simulink model "drives_project"  (R2023b)
settings: Solver=VariableStepAuto  StartTime=0.0  StopTime=0.1  RelTol=1e-3
InitFcn:
  | vm=220;
  | f=50;
  | P=2;
  | we=2*pi*f;
  | rs=0.1;
  | lls=0.06;
  | rr=0.1
  | llr=0.6;
  | lm=0.1;
  | lad=1/(1/lm+1/lls+1/llr);
  | laq=lad;
  | Tl=0.001;
  | B=0.0000;
  | J=0.00001;
libraries: spsVoltageMeasurementLib x9, spsSeriesRLCBranchLib x9, spsIGBTDiodeLib x6, simulink x3, spsDCVoltageSourceLib x1, sps_lib x1
settings Model: Creator=moham  LastModifiedBy=engyo
settings SolverCC: AlgebraicLoopSolver=TrustRegion
settings DebuggingCC: UnconnectedInputMsg=warning  UnconnectedOutputMsg=warning  UnconnectedLineMsg=warning
settings ModelReferenceCC: EnableRefExpFcnMdlSchedulingChecks=on

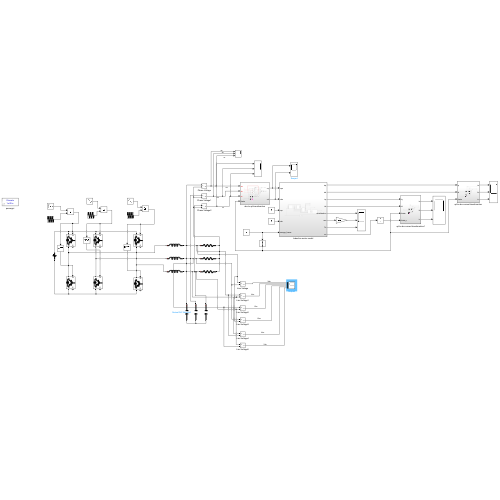
[thumbnail: Simulink's stored preview of the top-level diagram]
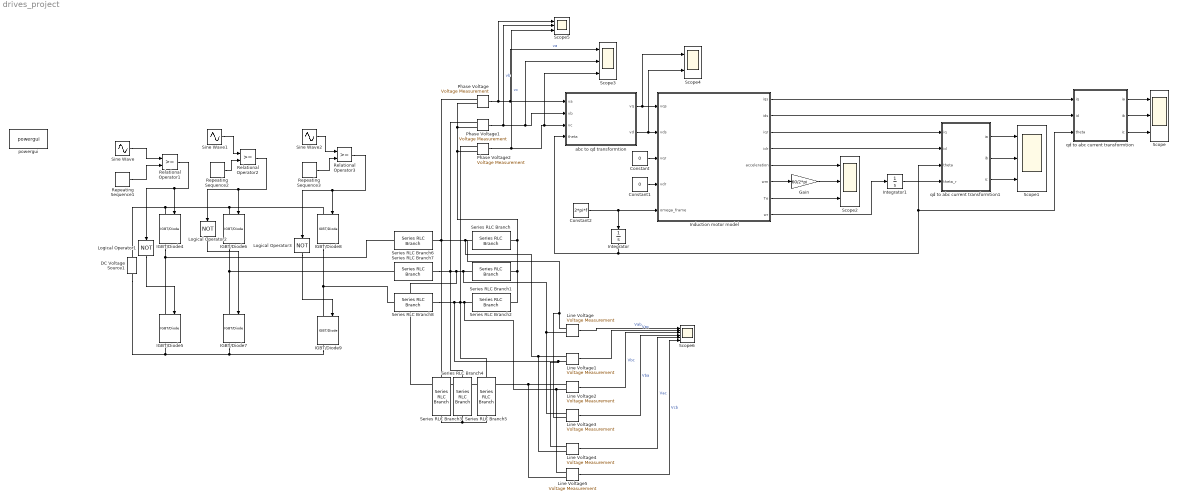
== system drives_project ==
  Constant : Constant  Value=0
  Constant1 : Constant  Value=0
  Constant2 : Constant  Value=2*pi*f
  DC Voltage Source1 : spsDCVoltageSourceLib/DC Voltage Source  Amplitude=100  Measurements=None
  Gain : Gain  Gain=60/2*pi
  IGBT/Diode{4..9} (6 alike) : spsIGBTDiodeLib/IGBT//Diode  Ron=1e-3  Rs=1e5  Cs=inf  Measurements=on
  Induction motor model : Subsystem
  Integrator : Integrator
  Integrator1 : Integrator
  Line Voltage{,1..5} (6 alike) : spsVoltageMeasurementLib/Voltage Measurement  PhasorSimulation=off  OutputType=Complex  PSBequivalent=0
  Logical Operator1 : Logic  Operator=NOT  AllPortsSameDT=off  OutDataTypeStr=boolean
  Logical Operator2 : Logic  Operator=NOT  AllPortsSameDT=off  OutDataTypeStr=boolean
  Logical Operator3 : Logic  Operator=NOT  AllPortsSameDT=off  OutDataTypeStr=boolean
  Phase Voltage : spsVoltageMeasurementLib/Voltage Measurement  PhasorSimulation=off  OutputType=Complex  PSBequivalent=0
  Phase Voltage1 : spsVoltageMeasurementLib/Voltage Measurement  PhasorSimulation=off  OutputType=Complex  PSBequivalent=0
  Phase Voltage2 : spsVoltageMeasurementLib/Voltage Measurement  PhasorSimulation=off  OutputType=Complex  PSBequivalent=0
  Relational Operator1 : RelationalOperator  OutDataTypeStr=boolean  RndMeth=Simplest  InputSameDT=off
  Relational Operator2 : RelationalOperator  OutDataTypeStr=boolean  RndMeth=Simplest  InputSameDT=off
  Relational Operator3 : RelationalOperator  OutDataTypeStr=boolean  RndMeth=Simplest  InputSameDT=off
  Repeating Sequence1 : simulink/Sources/Repeating Sequence  rep_seq_t=[0 (1/5050)/4 (1/5050)/2 (3/5050)/4 (1/5050)]  rep_seq_y=[0 1 0 -1 0]
  Repeating Sequence2 : simulink/Sources/Repeating Sequence  rep_seq_t=[0 (1/5050)/4 (1/5050)/2 (3/5050)/4 (1/5050)]  rep_seq_y=[0 1 0 -1 0]
  Repeating Sequence3 : simulink/Sources/Repeating Sequence  rep_seq_t=[0 (1/5050)/4 (1/5050)/2 (3/5050)/4 (1/5050)]  rep_seq_y=[0 1 0 -1 0]
  Scope{,1..3,5} (5 alike) : Scope  NumInputPorts=3
  Scope4 : Scope  NumInputPorts=2
  Scope6 : Scope  NumInputPorts=6
  Series RLC Branch : spsSeriesRLCBranchLib/Series RLC Branch  LConnTagsString=__new0  RConnTagsString=__new0  BranchType=R  Resistance=1  Inductance=1e-3  SetiL0=off  InitialCurrent=0  Capacitance=1e-6  Setx0=off  InitialVoltage=0  Measurements=None
  Series RLC Branch1 : spsSeriesRLCBranchLib/Series RLC Branch  LConnTagsString=__new0  RConnTagsString=__new0  BranchType=R  Resistance=1  Inductance=1e-3  SetiL0=off  InitialCurrent=0  Capacitance=1e-6  Setx0=off  InitialVoltage=0  Measurements=None
  Series RLC Branch2 : spsSeriesRLCBranchLib/Series RLC Branch  LConnTagsString=__new0  RConnTagsString=__new0  BranchType=R  Resistance=1  Inductance=1e-3  SetiL0=off  InitialCurrent=0  Capacitance=1e-6  Setx0=off  InitialVoltage=0  Measurements=None
  Series RLC Branch3 : spsSeriesRLCBranchLib/Series RLC Branch  LConnTagsString=__new0  RConnTagsString=__new0  BranchType=C  Resistance=1  Inductance=1e-3  SetiL0=off  InitialCurrent=0  Capacitance=100e-6  Setx0=off  InitialVoltage=0  Measurements=None
  Series RLC Branch4 : spsSeriesRLCBranchLib/Series RLC Branch  LConnTagsString=__new0  RConnTagsString=__new0  BranchType=C  Resistance=1  Inductance=1e-3  SetiL0=off  InitialCurrent=0  Capacitance=100e-6  Setx0=off  InitialVoltage=0  Measurements=None
  Series RLC Branch5 : spsSeriesRLCBranchLib/Series RLC Branch  LConnTagsString=__new0  RConnTagsString=__new0  BranchType=C  Resistance=1  Inductance=1e-3  SetiL0=off  InitialCurrent=0  Capacitance=100e-6  Setx0=off  InitialVoltage=0  Measurements=None
  Series RLC Branch6 : spsSeriesRLCBranchLib/Series RLC Branch  LConnTagsString=__new0  RConnTagsString=__new0  BranchType=L  Resistance=1  Inductance=1e-3  SetiL0=off  InitialCurrent=0  Capacitance=1e-6  Setx0=off  InitialVoltage=0  Measurements=None
  Series RLC Branch7 : spsSeriesRLCBranchLib/Series RLC Branch  LConnTagsString=__new0  RConnTagsString=__new0  BranchType=L  Resistance=1  Inductance=1e-3  SetiL0=off  InitialCurrent=0  Capacitance=1e-6  Setx0=off  InitialVoltage=0  Measurements=None
  Series RLC Branch8 : spsSeriesRLCBranchLib/Series RLC Branch  LConnTagsString=__new0  RConnTagsString=__new0  BranchType=L  Resistance=1  Inductance=1e-3  SetiL0=off  InitialCurrent=0  Capacitance=1e-6  Setx0=off  InitialVoltage=0  Measurements=None
  Sine Wave : Sin  Amplitude=0.95  Frequency=100*pi  SampleTime=0
  Sine Wave1 : Sin  Amplitude=0.95  Frequency=100*pi  Phase=(2*pi)/3  SampleTime=0
  Sine Wave2 : Sin  Amplitude=0.95  Frequency=100*pi  Phase=(4*pi)/3  SampleTime=0
  abc to qd transformtion : Subsystem
  powergui : sps_lib/powergui  Priority=1  SimulationMode=Discrete  SampleTime=10e-6  frequency=60  Iterations=50  frequencyindice=0  Pbase=100e6  ErrMax=1e-4  UnitsV=kV  UnitsW=MW  buscounter=0  FunctionMessages=off  echomessages=off  EnableUseOfTLC=off  CurrentSourceSwitches=off  DisableSnubberDevices=off  DisableRonSwitches=off  DisableVfSwitches=off  DisplayEquations=off  AutomaticDiscreteSolvers=off  SolverType=Tustin/Backward Euler (TBE)  Interpol=off  ExternalGateDelay=off  methode=off  Ts=100  x0status=blocks  SPID=on  SwTol=0  HookPort=off  NonlinearTolerance=1e-4  nMaxIteration=100  ContinueOnMaxIteration=off  RestoreLinks=warning  ResistiveCurrentMeasurement=off  Frange=[0:2:500]  Ylog=off  Xlog=on  ShowGrid=off  save=off  variable=ZData  structure=0  ZoomFFT=off  StartTime=0.0  cycles=1  DisplayStyle=1  fundamental=60  FreqAxis=off  MaxFrequency=1000  frequencyindicesteady=1  RmsSteady=1  display=off
  qd to abc current transformtion : Subsystem
  qd to abc current transformtion1 : Subsystem
  wires:
  abc to qd transformtion/2(vd) -> Scope4/2, Induction motor model/2(vds)
  abc to qd transformtion/1(vq) -> Scope4/1, Induction motor model/1(vqs)
  Induction motor model/1(iqs) -> qd to abc current transformtion/1(iq)
  Induction motor model/2(ids) -> qd to abc current transformtion/2(id)
  Induction motor model/3(iqr) -> qd to abc current transformtion1/1(iq)
  Induction motor model/4(idr) -> qd to abc current transformtion1/2(id)
  Constant1/1 -> Induction motor model/4(vdr)
  Constant/1 -> Induction motor model/3(vqr)
  Integrator/1 -> qd to abc current transformtion1/3(theta), qd to abc current transformtion/3(theta), abc to qd transformtion/4(theta)
  qd to abc current transformtion/1(ia) -> Scope/1
  qd to abc current transformtion/2(ib) -> Scope/2
  qd to abc current transformtion/3(ic) -> Scope/3
  qd to abc current transformtion1/1(ia) -> Scope1/1
  qd to abc current transformtion1/2(ib) -> Scope1/2
  qd to abc current transformtion1/3(ic) -> Scope1/3
  Induction motor model/8(wr) -> Integrator1/1
  Integrator1/1 -> qd to abc current transformtion1/4(theta_r)
  Constant2/1 -> Integrator/1, Induction motor model/5(omega_frame)
  Induction motor model/5(acceleration) -> Scope2/1
  Induction motor model/7(Te) -> Scope2/3
  Gain/1 -> Scope2/2
  Induction motor model/6(wm) -> Gain/1
  Repeating Sequence1/1 -> Relational Operator1/2
  Logical Operator2/1 -> IGBT/Diode7/1
  Logical Operator3/1 -> IGBT/Diode9/1
  Relational Operator1/1 -> Logical Operator1/1, IGBT/Diode4/1
  Repeating Sequence3/1 -> Relational Operator3/2
  Sine Wave/1 -> Relational Operator1/1
  Logical Operator1/1 -> IGBT/Diode5/1
  Relational Operator2/1 -> Logical Operator2/1, IGBT/Diode6/1
  Sine Wave2/1 -> Relational Operator3/1
  Sine Wave1/1 -> Relational Operator2/1
  Repeating Sequence2/1 -> Relational Operator2/2
  Relational Operator3/1 -> IGBT/Diode8/1, Logical Operator3/1
  Line Voltage/1 -> Scope6/1  "Vab"
  Phase Voltage/1 -> Scope5/1, Scope3/1, abc to qd transformtion/1(va)  "va"
  Phase Voltage1/1 -> Scope5/2, Scope3/2, abc to qd transformtion/2(vb)  "vb"
  Phase Voltage2/1 -> Scope5/3, Scope3/3, abc to qd transformtion/3(vc)  "vc"
  Line Voltage1/1 -> Scope6/2  "Vac"
  Line Voltage2/1 -> Scope6/3  "Vbc"
  Line Voltage3/1 -> Scope6/4  "Vba"
  Line Voltage4/1 -> Scope6/5  "Vac"
  Line Voltage5/1 -> Scope6/6  "Vcb"
  connections:
  IGBT/Diode8/RConn1 -- IGBT/Diode9/LConn1 -- Series RLC Branch8/LConn1
  IGBT/Diode6/RConn1 -- IGBT/Diode7/LConn1 -- Series RLC Branch7/LConn1
  DC Voltage Source1/RConn1 -- IGBT/Diode4/LConn1 -- IGBT/Diode8/LConn1 -- IGBT/Diode6/LConn1
  IGBT/Diode4/RConn1 -- IGBT/Diode5/LConn1 -- Series RLC Branch6/LConn1
  IGBT/Diode7/RConn1 -- IGBT/Diode9/RConn1 -- IGBT/Diode5/RConn1 -- DC Voltage Source1/LConn1
  Series RLC Branch/RConn1 -- Phase Voltage2/LConn2 -- Phase Voltage1/LConn2 -- Phase Voltage/LConn2 -- Series RLC Branch1/RConn1 -- Series RLC Branch2/RConn1
  Series RLC Branch6/RConn1 -- Phase Voltage/LConn1 -- Series RLC Branch3/LConn1 -- Line Voltage4/LConn2 -- Line Voltage1/LConn1 -- Line Voltage3/LConn2 -- Line Voltage/LConn1 -- Series RLC Branch/LConn1
  Series RLC Branch8/RConn1 -- Line Voltage4/LConn1 -- Line Voltage1/LConn2 -- Phase Voltage2/LConn1 -- Line Voltage5/LConn1 -- Line Voltage2/LConn2 -- Series RLC Branch2/LConn1 -- Series RLC Branch5/LConn1
  Series RLC Branch7/RConn1 -- Line Voltage5/LConn2 -- Line Voltage2/LConn1 -- Line Voltage3/LConn1 -- Line Voltage/LConn2 -- Series RLC Branch1/LConn1 -- Phase Voltage1/LConn1 -- Series RLC Branch4/LConn1
  Series RLC Branch3/RConn1 -- Series RLC Branch5/RConn1 -- Series RLC Branch4/RConn1

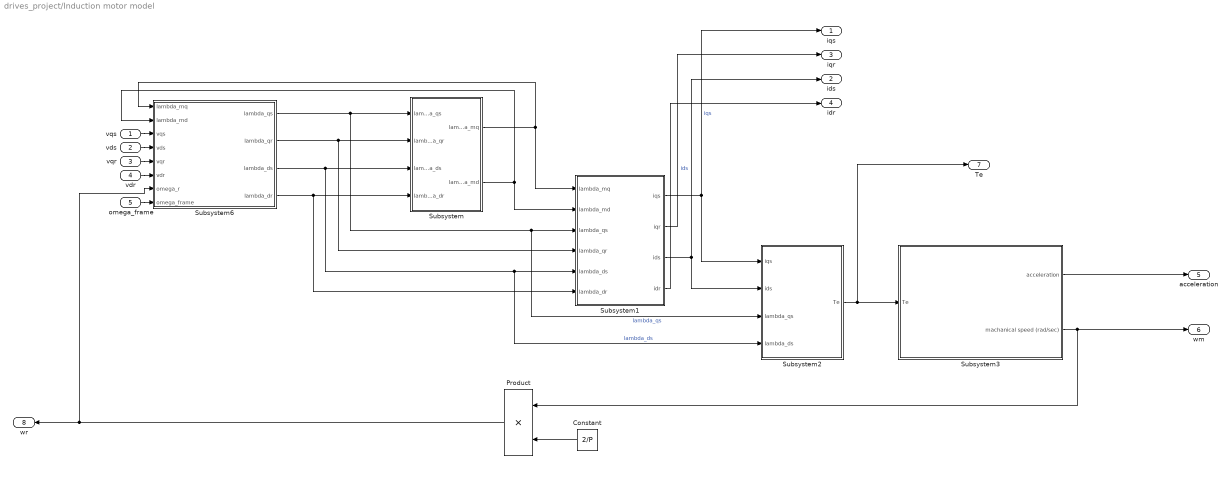
== system drives_project/Induction motor model ==
  vqs : Inport
  vds : Inport  Port=2
  vqr : Inport  Port=3
  vdr : Inport  Port=4
  omega_frame : Inport  Port=5
  Constant : Constant  Value=2/P
  Product : Product
  Subsystem : Subsystem
  Subsystem1 : Subsystem
  Subsystem2 : Subsystem
  Subsystem3 : Subsystem
  Subsystem6 : Subsystem
  iqs : Outport
  ids : Outport  Port=2
  iqr : Outport  Port=3
  idr : Outport  Port=4
  acceleration : Outport  Port=5
  wm : Outport  Port=6
  Te : Outport  Port=7
  wr : Outport  Port=8
  wires:
  Subsystem2/1(Te) -> Te/1, Subsystem3/1(Te)
  Subsystem6/3(lambda_ds) -> Subsystem2/4(lambda_ds), Subsystem1/5(lambda_ds), Subsystem/3(lambda_ds)  "lambda_ds"
  Subsystem/2(lambda_md) -> Subsystem1/2(lambda_md), Subsystem6/2(lambda_md)
  Subsystem1/4(idr) -> idr/1
  Subsystem1/2(iqr) -> iqr/1
  Subsystem/1(lambda_mq) -> Subsystem1/1(lambda_mq), Subsystem6/1(lambda_mq)
  Subsystem3/1(acceleration) -> acceleration/1
  Subsystem6/4(lambda_dr) -> Subsystem1/6(lambda_dr), Subsystem/4(lambda_dr)
  Subsystem6/1(lambda_qs) -> Subsystem2/3(lambda_qs), Subsystem1/3(lambda_qs), Subsystem/1(lambda_qs)  "lambda_qs"
  Subsystem1/3(ids) -> ids/1, Subsystem2/2(ids)  "ids"
  Subsystem6/2(lambda_qr) -> Subsystem1/4(lambda_qr), Subsystem/2(lambda_qr)
  vqr/1 -> Subsystem6/5(vqr)
  Subsystem3/2(machanical speed (rad/sec)) -> wm/1, Product/1
  Subsystem1/1(iqs) -> iqs/1, Subsystem2/1(iqs)  "iqs"
  vdr/1 -> Subsystem6/6(vdr)
  vds/1 -> Subsystem6/4(vds)
  Constant/1 -> Product/2
  Product/1 -> wr/1, Subsystem6/7(omega_r)
  vqs/1 -> Subsystem6/3(vqs)
  omega_frame/1 -> Subsystem6/8(omega_frame)

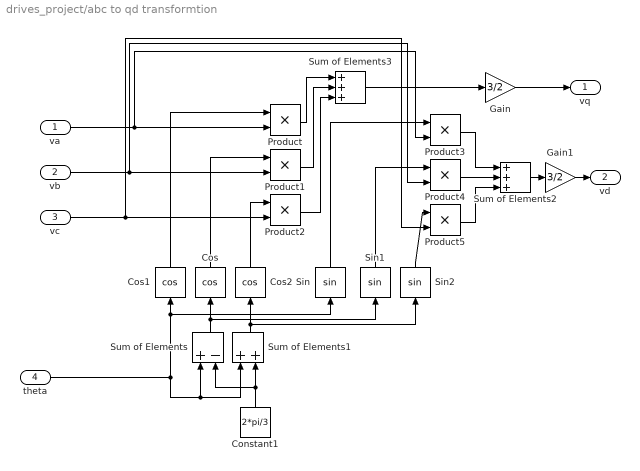
== system drives_project/abc to qd transformtion ==
  va : Inport
  vb : Inport  Port=2
  vc : Inport  Port=3
  theta : Inport  Port=4
  Constant1 : Constant  Value=2*pi/3
  Cos : Trigonometry  Operator=cos
  Cos1 : Trigonometry  Operator=cos
  Cos2 : Trigonometry  Operator=cos
  Gain : Gain  Gain=3/2
  Gain1 : Gain  Gain=3/2
  Product{,1..5} (6 alike) : Product
  Sin : Trigonometry
  Sin1 : Trigonometry
  Sin2 : Trigonometry
  Sum of Elements : Sum  Inputs=+-
  Sum of Elements1 : Sum
  Sum of Elements2 : Sum  Inputs=+++
  Sum of Elements3 : Sum  Inputs=+++
  vq : Outport
  vd : Outport  Port=2
  wires:
  vc/1 -> Product2/2, Product5/2
  theta/1 -> Sum of Elements1/1, Sum of Elements/1, Sin/1, Cos1/1
  va/1 -> Product3/2, Product/2
  vb/1 -> Product1/2, Product4/2
  Cos/1 -> Product1/1
  Constant1/1 -> Sum of Elements1/2, Sum of Elements/2
  Cos1/1 -> Product/1
  Product/1 -> Sum of Elements3/1
  Sin/1 -> Product3/1
  Product1/1 -> Sum of Elements3/2
  Sum of Elements/1 -> Sin1/1, Cos/1
  Sin2/1 -> Product5/1
  Product5/1 -> Sum of Elements2/3
  Sum of Elements3/1 -> Gain/1
  Sum of Elements1/1 -> Sin2/1, Cos2/1
  Product3/1 -> Sum of Elements2/1
  Product4/1 -> Sum of Elements2/2
  Product2/1 -> Sum of Elements3/3
  Cos2/1 -> Product2/1
  Sin1/1 -> Product4/1
  Gain/1 -> vq/1
  Gain1/1 -> vd/1
  Sum of Elements2/1 -> Gain1/1

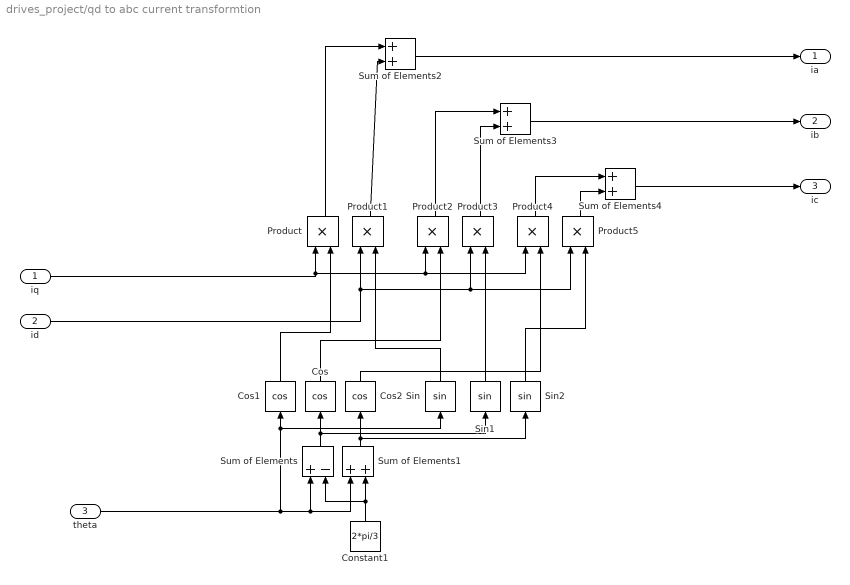
== system drives_project/qd to abc current transformtion ==
  iq : Inport
  id : Inport  Port=2
  theta : Inport  Port=3
  Constant1 : Constant  Value=2*pi/3
  Cos : Trigonometry  Operator=cos
  Cos1 : Trigonometry  Operator=cos
  Cos2 : Trigonometry  Operator=cos
  Product{,1..5} (6 alike) : Product
  Sin : Trigonometry
  Sin1 : Trigonometry
  Sin2 : Trigonometry
  Sum of Elements : Sum  Inputs=+-
  Sum of Elements{1..4} (4 alike) : Sum
  ia : Outport
  ib : Outport  Port=2
  ic : Outport  Port=3
  wires:
  theta/1 -> Sin/1, Cos1/1, Sum of Elements1/1, Sum of Elements/1
  Constant1/1 -> Sum of Elements1/2, Sum of Elements/2
  Sum of Elements/1 -> Sin1/1, Cos/1
  Sum of Elements1/1 -> Sin2/1, Cos2/1
  iq/1 -> Product2/1, Product4/1, Product/1
  Cos1/1 -> Product/2
  id/1 -> Product1/1, Product3/1, Product5/1
  Sin/1 -> Product1/2
  Cos/1 -> Product2/2
  Sin1/1 -> Product3/2
  Cos2/1 -> Product4/2
  Sin2/1 -> Product5/2
  Product1/1 -> Sum of Elements2/2
  Product/1 -> Sum of Elements2/1
  Product3/1 -> Sum of Elements3/2
  Product2/1 -> Sum of Elements3/1
  Product5/1 -> Sum of Elements4/2
  Product4/1 -> Sum of Elements4/1
  Sum of Elements2/1 -> ia/1
  Sum of Elements3/1 -> ib/1
  Sum of Elements4/1 -> ic/1

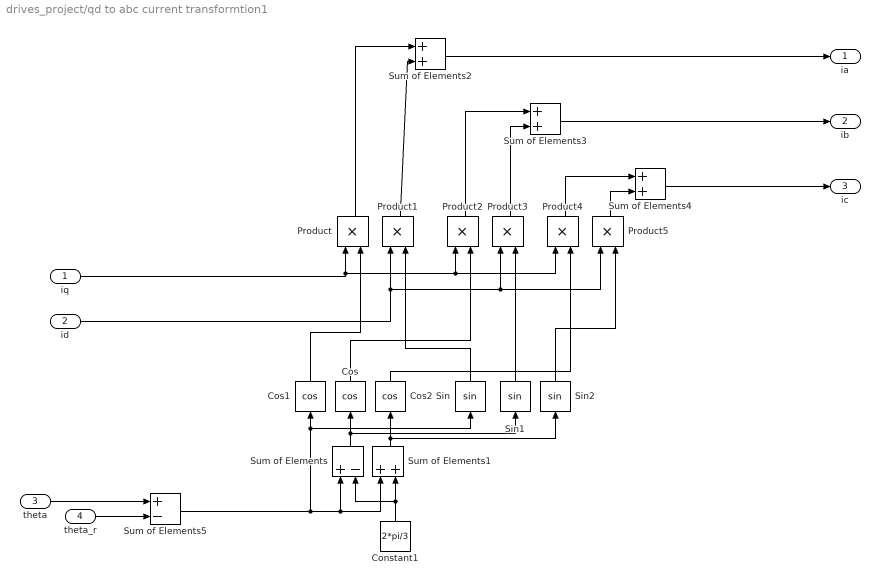
== system drives_project/qd to abc current transformtion1 ==
  iq : Inport
  id : Inport  Port=2
  theta : Inport  Port=3
  theta_r : Inport  Port=4
  Constant1 : Constant  Value=2*pi/3
  Cos : Trigonometry  Operator=cos
  Cos1 : Trigonometry  Operator=cos
  Cos2 : Trigonometry  Operator=cos
  Product{,1..5} (6 alike) : Product
  Sin : Trigonometry
  Sin1 : Trigonometry
  Sin2 : Trigonometry
  Sum of Elements : Sum  Inputs=+-
  Sum of Elements{1..4} (4 alike) : Sum
  Sum of Elements5 : Sum  Inputs=+-
  ia : Outport
  ib : Outport  Port=2
  ic : Outport  Port=3
  wires:
  Sum of Elements5/1 -> Sin/1, Cos1/1, Sum of Elements1/1, Sum of Elements/1
  Constant1/1 -> Sum of Elements1/2, Sum of Elements/2
  Sum of Elements/1 -> Sin1/1, Cos/1
  Sum of Elements1/1 -> Sin2/1, Cos2/1
  iq/1 -> Product2/1, Product4/1, Product/1
  Cos1/1 -> Product/2
  id/1 -> Product1/1, Product3/1, Product5/1
  Sin/1 -> Product1/2
  Cos/1 -> Product2/2
  Sin1/1 -> Product3/2
  Cos2/1 -> Product4/2
  Sin2/1 -> Product5/2
  Product1/1 -> Sum of Elements2/2
  Product/1 -> Sum of Elements2/1
  Product3/1 -> Sum of Elements3/2
  Product2/1 -> Sum of Elements3/1
  Product5/1 -> Sum of Elements4/2
  Product4/1 -> Sum of Elements4/1
  Sum of Elements2/1 -> ia/1
  Sum of Elements3/1 -> ib/1
  Sum of Elements4/1 -> ic/1
  theta_r/1 -> Sum of Elements5/2
  theta/1 -> Sum of Elements5/1

== system drives_project/Induction motor model/Subsystem ==
  lambda_qs : Inport
  lambda_qr : Inport  Port=2
  lambda_ds : Inport  Port=3
  lambda_dr : Inport  Port=4
  Subsystem4 : Subsystem
  Subsystem5 : Subsystem
  lambda_mq : Outport
  lambda_md : Outport  Port=2
  wires:
  lambda_ds/1 -> Subsystem5/1(lambda_ds)
  Subsystem5/1(lambda_md) -> lambda_md/1
  lambda_qr/1 -> Subsystem4/2(lambda_qr)
  Subsystem4/1(lambda_mq) -> lambda_mq/1
  lambda_qs/1 -> Subsystem4/1(lambda_qs)
  lambda_dr/1 -> Subsystem5/2(lambda_dr)

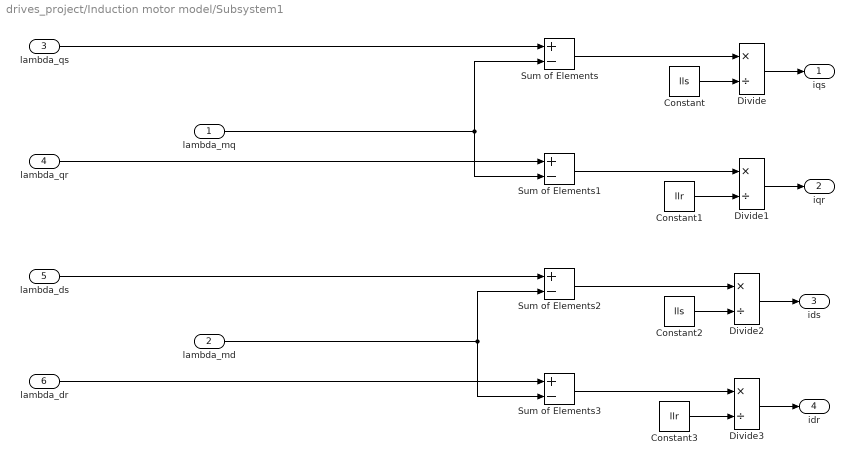
== system drives_project/Induction motor model/Subsystem1 ==
  lambda_mq : Inport
  lambda_md : Inport  Port=2
  lambda_qs : Inport  Port=3
  lambda_qr : Inport  Port=4
  lambda_ds : Inport  Port=5
  lambda_dr : Inport  Port=6
  Constant : Constant  Value=lls
  Constant1 : Constant  Value=llr
  Constant2 : Constant  Value=lls
  Constant3 : Constant  Value=llr
  Divide{,1..3} (4 alike) : Product  Inputs=*/
  Sum of Elements{,1..3} (4 alike) : Sum  Inputs=+-
  iqs : Outport
  iqr : Outport  Port=2
  ids : Outport  Port=3
  idr : Outport  Port=4
  wires:
  lambda_mq/1 -> Sum of Elements/2, Sum of Elements1/2
  Constant/1 -> Divide/2
  lambda_qs/1 -> Sum of Elements/1
  Divide/1 -> iqs/1
  Divide2/1 -> ids/1
  lambda_qr/1 -> Sum of Elements1/1
  Divide1/1 -> iqr/1
  lambda_md/1 -> Sum of Elements2/2, Sum of Elements3/2
  Sum of Elements/1 -> Divide/1
  Constant1/1 -> Divide1/2
  Sum of Elements1/1 -> Divide1/1
  Constant3/1 -> Divide3/2
  Constant2/1 -> Divide2/2
  Divide3/1 -> idr/1
  lambda_ds/1 -> Sum of Elements2/1
  Sum of Elements2/1 -> Divide2/1
  Sum of Elements3/1 -> Divide3/1
  lambda_dr/1 -> Sum of Elements3/1

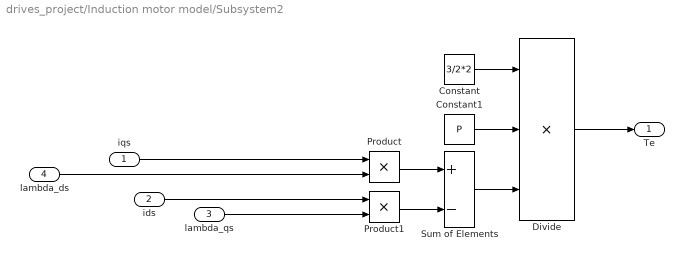
== system drives_project/Induction motor model/Subsystem2 ==
  iqs : Inport
  ids : Inport  Port=2
  lambda_qs : Inport  Port=3
  lambda_ds : Inport  Port=4
  Constant : Constant  Value=3/2*2
  Constant1 : Constant  Value=P
  Divide : Product  Inputs=***
  Product : Product
  Product1 : Product
  Sum of Elements : Sum  Inputs=+-
  Te : Outport
  wires:
  lambda_qs/1 -> Product1/2
  Product1/1 -> Sum of Elements/2
  Constant1/1 -> Divide/2
  Divide/1 -> Te/1
  iqs/1 -> Product/1
  Product/1 -> Sum of Elements/1
  Constant/1 -> Divide/1
  Sum of Elements/1 -> Divide/3
  lambda_ds/1 -> Product/2
  ids/1 -> Product1/1

== system drives_project/Induction motor model/Subsystem3 ==
  Te : Inport
  Constant : Constant  Value=Tl
  Constant1 : Constant  Value=B
  Constant2 : Constant  Value=J
  Divide : Product  Inputs=*/
  Integrator : Integrator
  Product : Product
  Sum of Elements : Sum  Inputs=+--
  acceleration : Outport
  machanical speed (rad/sec) : Outport  Port=2
  wires:
  Constant2/1 -> Divide/2
  Integrator/1 -> machanical speed (rad/sec)/1, Product/2
  Constant1/1 -> Product/1
  Product/1 -> Sum of Elements/3
  Divide/1 -> acceleration/1, Integrator/1
  Sum of Elements/1 -> Divide/1
  Constant/1 -> Sum of Elements/2
  Te/1 -> Sum of Elements/1

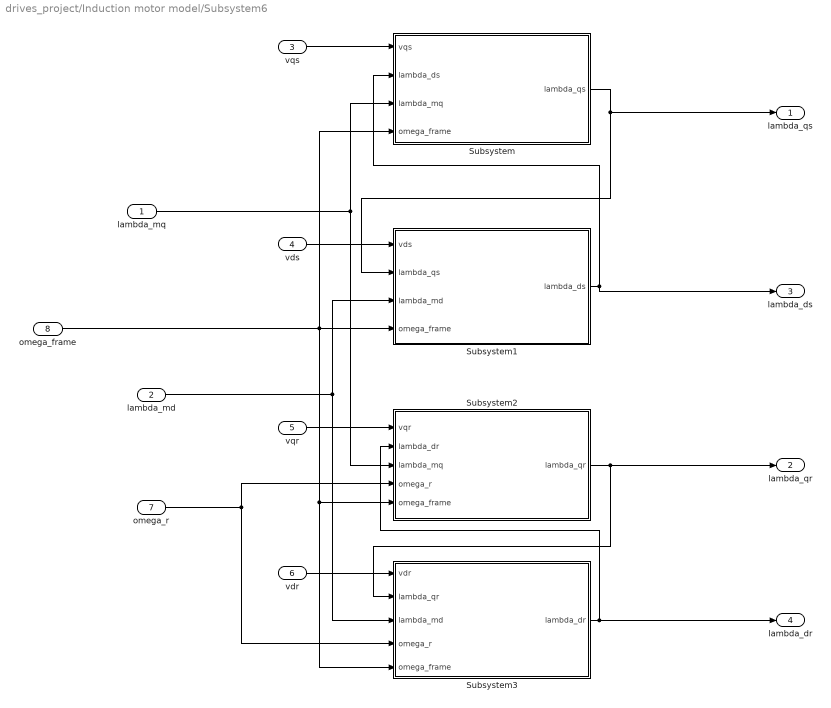
== system drives_project/Induction motor model/Subsystem6 ==
  lambda_mq : Inport
  lambda_md : Inport  Port=2
  vqs : Inport  Port=3
  vds : Inport  Port=4
  vqr : Inport  Port=5
  vdr : Inport  Port=6
  omega_r : Inport  Port=7
  omega_frame : Inport  Port=8
  Subsystem : Subsystem
  Subsystem1 : Subsystem
  Subsystem2 : Subsystem
  Subsystem3 : Subsystem
  lambda_qs : Outport
  lambda_qr : Outport  Port=2
  lambda_ds : Outport  Port=3
  lambda_dr : Outport  Port=4
  wires:
  Subsystem3/1(lambda_dr) -> Subsystem2/2(lambda_dr), lambda_dr/1
  lambda_md/1 -> Subsystem1/3(lambda_md), Subsystem3/3(lambda_md)
  Subsystem/1(lambda_qs) -> lambda_qs/1, Subsystem1/2(lambda_qs)
  Subsystem2/1(lambda_qr) -> Subsystem3/2(lambda_qr), lambda_qr/1
  Subsystem1/1(lambda_ds) -> lambda_ds/1, Subsystem/2(lambda_ds)
  vqr/1 -> Subsystem2/1(vqr)
  vds/1 -> Subsystem1/1(vds)
  lambda_mq/1 -> Subsystem2/3(lambda_mq), Subsystem/3(lambda_mq)
  vdr/1 -> Subsystem3/1(vdr)
  omega_r/1 -> Subsystem3/4(omega_r), Subsystem2/4(omega_r)
  vqs/1 -> Subsystem/1(vqs)
  omega_frame/1 -> Subsystem2/5(omega_frame), Subsystem3/5(omega_frame), Subsystem/4(omega_frame), Subsystem1/4(omega_frame)

== system drives_project/Induction motor model/Subsystem/Subsystem4 ==
  lambda_qs : Inport
  lambda_qr : Inport  Port=2
  Constant : Constant  Value=lls
  Constant1 : Constant  Value=llr
  Constant2 : Constant  Value=laq
  Divide : Product  Inputs=*/
  Divide1 : Product  Inputs=*/
  Product : Product
  Sum of Elements : Sum
  lambda_mq : Outport
  wires:
  Divide/1 -> Sum of Elements/1
  Constant2/1 -> Product/2
  lambda_qs/1 -> Divide/1
  Constant/1 -> Divide/2
  Constant1/1 -> Divide1/2
  Sum of Elements/1 -> Product/1
  Divide1/1 -> Sum of Elements/2
  lambda_qr/1 -> Divide1/1
  Product/1 -> lambda_mq/1

== system drives_project/Induction motor model/Subsystem/Subsystem5 ==
  lambda_ds : Inport
  lambda_dr : Inport  Port=2
  Constant : Constant  Value=lls
  Constant1 : Constant  Value=llr
  Constant2 : Constant  Value=lad
  Divide : Product  Inputs=*/
  Divide1 : Product  Inputs=*/
  Product : Product
  Sum of Elements : Sum
  lambda_md : Outport
  wires:
  Divide/1 -> Sum of Elements/1
  Constant2/1 -> Product/2
  lambda_ds/1 -> Divide/1
  Constant/1 -> Divide/2
  Constant1/1 -> Divide1/2
  Sum of Elements/1 -> Product/1
  Divide1/1 -> Sum of Elements/2
  lambda_dr/1 -> Divide1/1
  Product/1 -> lambda_md/1

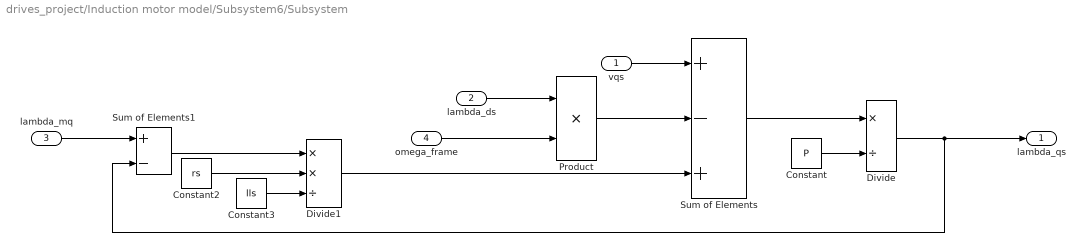
== system drives_project/Induction motor model/Subsystem6/Subsystem ==
  vqs : Inport
  lambda_ds : Inport  Port=2
  lambda_mq : Inport  Port=3
  omega_frame : Inport  Port=4
  Constant : Constant  Value=P
  Constant2 : Constant  Value=rs
  Constant3 : Constant  Value=lls
  Divide : Product  Inputs=*/
  Divide1 : Product  Inputs=**/
  Product : Product
  Sum of Elements : Sum  Inputs=+-+
  Sum of Elements1 : Sum  Inputs=+-
  lambda_qs : Outport
  wires:
  Constant2/1 -> Divide1/2
  Sum of Elements/1 -> Divide/1
  Sum of Elements1/1 -> Divide1/1
  omega_frame/1 -> Product/2
  Divide/1 -> lambda_qs/1, Sum of Elements1/2
  Constant/1 -> Divide/2
  lambda_ds/1 -> Product/1
  vqs/1 -> Sum of Elements/1
  Product/1 -> Sum of Elements/2
  lambda_mq/1 -> Sum of Elements1/1
  Divide1/1 -> Sum of Elements/3
  Constant3/1 -> Divide1/3

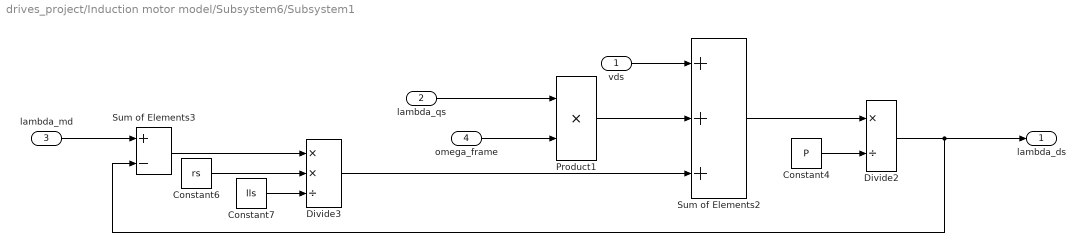
== system drives_project/Induction motor model/Subsystem6/Subsystem1 ==
  vds : Inport
  lambda_qs : Inport  Port=2
  lambda_md : Inport  Port=3
  omega_frame : Inport  Port=4
  Constant4 : Constant  Value=P
  Constant6 : Constant  Value=rs
  Constant7 : Constant  Value=lls
  Divide2 : Product  Inputs=*/
  Divide3 : Product  Inputs=**/
  Product1 : Product
  Sum of Elements2 : Sum  Inputs=+++
  Sum of Elements3 : Sum  Inputs=+-
  lambda_ds : Outport
  wires:
  vds/1 -> Sum of Elements2/1
  Constant4/1 -> Divide2/2
  Sum of Elements3/1 -> Divide3/1
  Constant7/1 -> Divide3/3
  Divide2/1 -> lambda_ds/1, Sum of Elements3/2
  lambda_md/1 -> Sum of Elements3/1
  Divide3/1 -> Sum of Elements2/3
  Sum of Elements2/1 -> Divide2/1
  Constant6/1 -> Divide3/2
  Product1/1 -> Sum of Elements2/2
  omega_frame/1 -> Product1/2
  lambda_qs/1 -> Product1/1

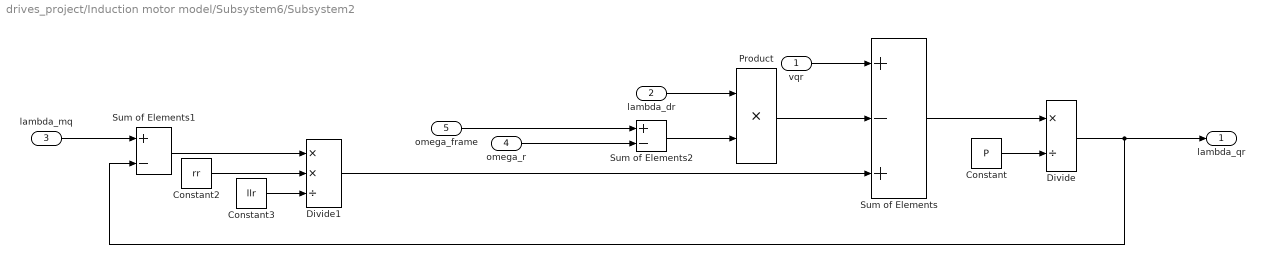
== system drives_project/Induction motor model/Subsystem6/Subsystem2 ==
  vqr : Inport
  lambda_dr : Inport  Port=2
  lambda_mq : Inport  Port=3
  omega_r : Inport  Port=4
  omega_frame : Inport  Port=5
  Constant : Constant  Value=P
  Constant2 : Constant  Value=rr
  Constant3 : Constant  Value=llr
  Divide : Product  Inputs=*/
  Divide1 : Product  Inputs=**/
  Product : Product
  Sum of Elements : Sum  Inputs=+-+
  Sum of Elements1 : Sum  Inputs=+-
  Sum of Elements2 : Sum  Inputs=+-
  lambda_qr : Outport
  wires:
  Constant2/1 -> Divide1/2
  Sum of Elements/1 -> Divide/1
  Sum of Elements1/1 -> Divide1/1
  Divide/1 -> lambda_qr/1, Sum of Elements1/2
  Constant/1 -> Divide/2
  lambda_dr/1 -> Product/1
  vqr/1 -> Sum of Elements/1
  Product/1 -> Sum of Elements/2
  lambda_mq/1 -> Sum of Elements1/1
  Divide1/1 -> Sum of Elements/3
  Constant3/1 -> Divide1/3
  Sum of Elements2/1 -> Product/2
  omega_frame/1 -> Sum of Elements2/1
  omega_r/1 -> Sum of Elements2/2

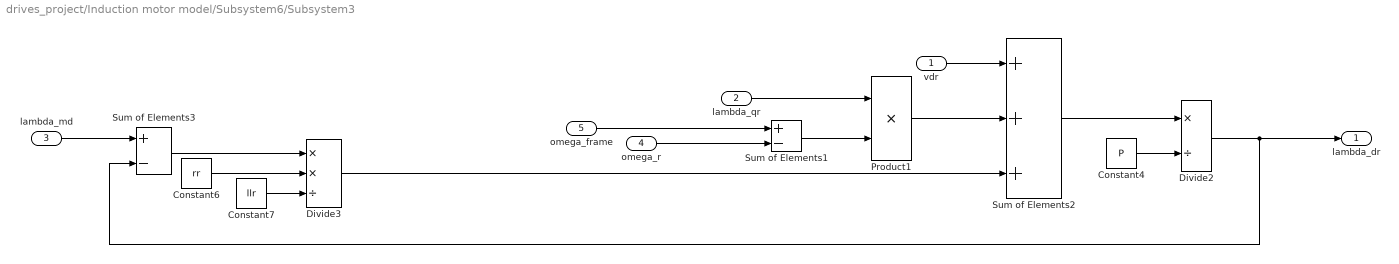
== system drives_project/Induction motor model/Subsystem6/Subsystem3 ==
  vdr : Inport
  lambda_qr : Inport  Port=2
  lambda_md : Inport  Port=3
  omega_r : Inport  Port=4
  omega_frame : Inport  Port=5
  Constant4 : Constant  Value=P
  Constant6 : Constant  Value=rr
  Constant7 : Constant  Value=llr
  Divide2 : Product  Inputs=*/
  Divide3 : Product  Inputs=**/
  Product1 : Product
  Sum of Elements1 : Sum  Inputs=+-
  Sum of Elements2 : Sum  Inputs=+++
  Sum of Elements3 : Sum  Inputs=+-
  lambda_dr : Outport
  wires:
  vdr/1 -> Sum of Elements2/1
  Constant4/1 -> Divide2/2
  Sum of Elements3/1 -> Divide3/1
  Constant7/1 -> Divide3/3
  Divide2/1 -> lambda_dr/1, Sum of Elements3/2
  lambda_md/1 -> Sum of Elements3/1
  Divide3/1 -> Sum of Elements2/3
  Sum of Elements2/1 -> Divide2/1
  Constant6/1 -> Divide3/2
  Product1/1 -> Sum of Elements2/2
  lambda_qr/1 -> Product1/1
  omega_frame/1 -> Sum of Elements1/1
  omega_r/1 -> Sum of Elements1/2
  Sum of Elements1/1 -> Product1/2
